simulink model "DOB_ros"  (R2017b)
settings: Solver=FixedStepAuto  StartTime=0.0  StopTime=inf  FixedStep=dt_ros  RelTol=1e-3
values from neighbouring files (symbols this model uses):
  a1 = @(vx, dphi) [0, 0, 0, 1]    [DOB_ros_adaptive_setup.m]    (also in DOB_ros_adaptive_w_kappa_setup.m = init)
  a2 = @(vx, dphi) [vx/cos(dphi)^2, 0, 1, ds]    [DOB_ros_adaptive_setup.m]    (also in DOB_ros_adaptive_w_kappa_setup.m = init)
  a3 = @(vx, dphi) [0, 0, -(Caf+Car)/(m*vx), -vx-(Caf*a-Car*b)/(m*vx)]    [DOB_ros_adaptive_setup.m]    (also in DOB_ros_adaptive_w_kappa_setup.m = init)
  b0 = init    [DOB_ros_adaptive_w_kappa_setup.m]
  b1 = init    [DOB_ros_adaptive_w_kappa_setup.m]    (also in DOB_ros_setup.m = 107.91)
  b2 = init    [DOB_ros_adaptive_w_kappa_setup.m]    (also in DOB_ros_setup.m = 71.28)
  b3 = Caf / m    (= 107.91)    [DOB_ros_adaptive_setup.m]    (also in DOB_ros_adaptive_w_kappa_setup.m = init)
  b4 = a * Caf / Iz    (= 71.28)    [DOB_ros_adaptive_setup.m]    (also in DOB_ros_adaptive_w_kappa_setup.m = init)
  b5 = init    [DOB_ros_adaptive_w_kappa_setup.m]
  Dd = single([Numc{1}(3:end) 0 0]/Numc{1}(3))    [DOB_ros_adaptive_setup.m]    (also in DOB_ros_adaptive_w_kappa_setup.m; DOB_ros_setup.m)
  Dn = single(Denc{1}/Numc{1}(3))    [DOB_ros_adaptive_setup.m]    (also in DOB_ros_adaptive_w_kappa_setup.m; DOB_ros_setup.m)
  dphi_list = -1:0.1:1    [DOB_ros_adaptive_w_kappa_setup.m]
  dt_ros = 0.02    [DOB_ros_adaptive_setup.m]    (also in DOB_ros_adaptive_w_kappa_setup.m; DOB_ros_setup.m)
  dt_ros_single = single(0.02)    [DOB_ros_adaptive_setup.m]    (also in DOB_ros_adaptive_w_kappa_setup.m; DOB_ros_setup.m)
  kappa_list = -0.02:0.005:0.02    [DOB_ros_adaptive_w_kappa_setup.m]
  kc11 = single(0.3)    [DOB_ros_adaptive_setup.m]    (also in DOB_ros_adaptive_w_kappa_setup.m = single(1); DOB_ros_setup.m = kc1)
  kc12 = single(1)    [DOB_ros_adaptive_setup.m]    (also in DOB_ros_adaptive_w_kappa_setup.m = single(0); DOB_ros_setup.m = 1)
  kc2 = single(0.25)    [DOB_ros_adaptive_setup.m]    (also in DOB_ros_adaptive_w_kappa_setup.m = single(0.5); DOB_ros_setup.m = single(0.1))
  steering_ratio = 14.8    [DOB_ros_adaptive_setup.m]    (also in DOB_ros_adaptive_w_kappa_setup.m; DOB_ros_setup.m)
  v_list = 1:0.2:20    [DOB_ros_adaptive_w_kappa_setup.m]
undefined symbols (not defined in the file or in its folder): DCancel, DEst, DQ, Enable, NQ, SteeringWheelAngleCmd, SteeringWheelAngleVelocity
libraries: robotlib x6, cstblocks x1
settings Model: Creator=chen_tang  LastModifiedBy=root
settings OptimizationCC: PassReuseOutputArgsThreshold=0  MaxStackSize=64
settings DebuggingCC: ParameterTunabilityLossMsg=error
settings HardwareCC: ProdBitPerPointer=32  ProdBitPerSizeT=32  ProdBitPerPtrDiffT=32  ProdLargestAtomicFloat=None  ProdIntDivRoundTo=Undefined  ProdEndianess=Unspecified  ProdWordSize=32  ProdHWDeviceType=Generic->Unspecified (assume 32-bit Generic)  UseEmbeddedCoderFeatures=off
settings SFSimCC: MATLABDynamicMemAlloc=off
settings RTWCC: SystemTargetFile=ert.tlc  HardwareBoard=Robot Operating System (ROS)  TemplateMakefile=ert_default_tmf  GenerateReport=on  Toolchain=Catkin  LaunchReport=on  TargetLang=C++
settings CodeAppCC: ForceParamTrailComments=on  OperatorAnnotations=on  StateflowObjectComments=on  MATLABSourceComments=on
settings ERTTargetCC: ERTCustomFileBanners=off  SupportContinuousTime=on  SupportNonInlinedSFcns=on  RemoveResetFunc=off  ModelStepFunctionPrototypeControlCompliant=off

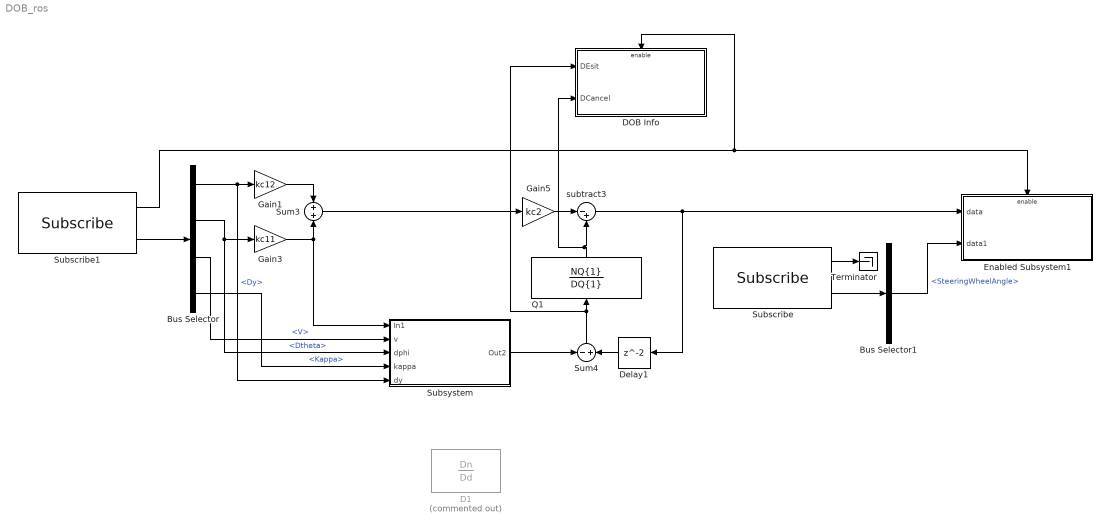
== system DOB_ros ==
  Bus Selector : BusSelector  OutputSignals=Dy,Dtheta,V,Kappa
  Bus Selector1 : BusSelector  OutputSignals=SteeringWheelAngle
  D1 : DiscreteTransferFcn  Commented=on  Numerator=Dn  Denominator=Dd  SampleTime=dt_ros
  DOB Info : Subsystem  TreatAsAtomicUnit=on
  Delay1 : Delay  InitialCondition=0  SampleTime=dt_ros
  Enabled Subsystem1 : Subsystem  TreatAsAtomicUnit=on
  Gain1 : Gain  Gain=kc12  OutDataTypeStr=single
  Gain3 : Gain  Gain=kc11  OutDataTypeStr=single
  Gain5 : Gain  Gain=kc2
  Q1 : DiscreteTransferFcn  Numerator=NQ{1}  Denominator=DQ{1}  SampleTime=dt_ros
  Subscribe : robotlib/Subscribe  SourceLibraryInfo=This block requires Robotics System Toolbox  topicSource=Specify your own  topic=/vehicle/steering_report  messageType=dbw_mkz_msgs/SteeringReport  sampleTime=-1  messageQueueLength=1
      settings: SourceProductBaseCode=RO
  Subscribe1 : robotlib/Subscribe  SourceLibraryInfo=This block requires Robotics System Toolbox  topicSource=Specify your own  topic=/tracking_info  messageType=controller/TrackingInfo  sampleTime=-1  messageQueueLength=1
      link override SourceBlock: ROSTopic=/tracking_info  ROSMessageType=controller/TrackingInfo  SLBusName=SL_Bus_DOB_ros_controller_TrackingInfo  ModelName=DOB_ros  BlockId=Sub_DOB_ros_174
      settings: SourceProductBaseCode=RO
  Subsystem : Subsystem
  Sum3 : Sum  Inputs=+|+  AccumDataTypeStr=single  OutDataTypeStr=single
  Sum4 : Sum  Inputs=-|+
  Terminator : Terminator
  subtract3 : Sum  Inputs=|-+  AccumDataTypeStr=single
  wires:
  Subscribe1/2 -> Bus Selector/1
  Gain3/1 -> Sum3/2, Subsystem/1(In1)
  Subscribe1/1 -> DOB Info/Enable, Enabled Subsystem1/Enable
  Bus Selector/2 -> Subsystem/3(dphi), Gain3/1  "<Dtheta>"
  Gain5/1 -> subtract3/1
  subtract3/1 -> Delay1/1, Enabled Subsystem1/1(data)
  Sum3/1 -> Gain5/1
  Subscribe/1 -> Terminator/1
  Subscribe/2 -> Bus Selector1/1
  Bus Selector1/1 -> Enabled Subsystem1/2(data1)  "<SteeringWheelAngle>"
  Delay1/1 -> Sum4/2
  Sum4/1 -> DOB Info/1(DEsit), Q1/1
  Subsystem/1(Out2) -> Sum4/1
  Q1/1 -> subtract3/2, DOB Info/2(DCancel)
  Bus Selector/1 -> Subsystem/5(dy), Gain1/1  "<Dy>"
  Gain1/1 -> Sum3/1
  Bus Selector/3 -> Subsystem/2(v)  "<V>"
  Bus Selector/4 -> Subsystem/4("kappa ")  "<Kappa>"

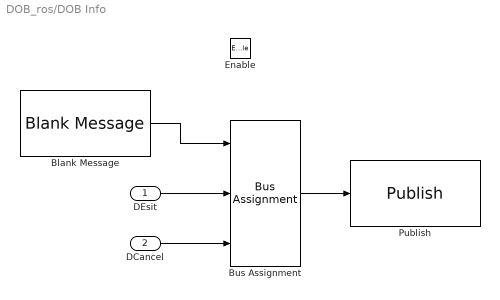
== system DOB_ros/DOB Info ==
  DEsit : Inport
  DCancel : Inport  Port=2
  Enable : EnablePort
  Blank Message : robotlib/Blank Message  SourceLibraryInfo=This block requires Robotics System Toolbox  messageType=controller/DobInfo  SampleTime=dt_ros
      settings: SourceProductBaseCode=RO
  Bus Assignment : BusAssignment  AssignedSignals=DEst,DCancel
  Publish : robotlib/Publish  SourceLibraryInfo=This block requires Robotics System Toolbox  topicSource=Specify your own  topic=/dob_info  messageType=controller/DobInfo  messageQueueLength=1
      settings: SourceProductBaseCode=RO
  wires:
  Bus Assignment/1 -> Publish/1
  Blank Message/1 -> Bus Assignment/1
  DEsit/1 -> Bus Assignment/2
  DCancel/1 -> Bus Assignment/3

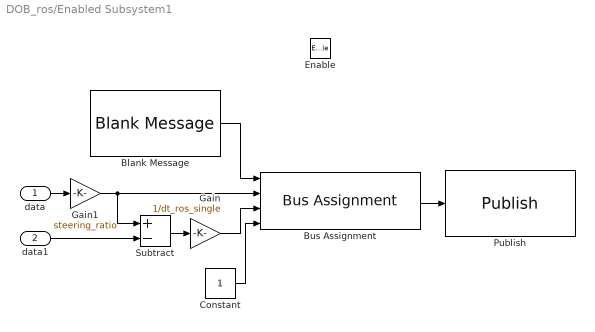
== system DOB_ros/Enabled Subsystem1 ==
  data : Inport  OutDataTypeStr=single
  data1 : Inport  Port=2  OutDataTypeStr=single
  Enable : EnablePort
  Blank Message : robotlib/Blank Message  SourceLibraryInfo=This block requires Robotics System Toolbox  messageType=dbw_mkz_msgs/SteeringCmd  SampleTime=dt_ros
      settings: SourceProductBaseCode=RO
  Bus Assignment : BusAssignment  AssignedSignals=SteeringWheelAngleCmd,SteeringWheelAngleVelocity,Enable
  Constant : Constant  OutDataTypeStr=boolean
  Gain : Gain  Gain=1/dt_ros_single  ParamDataTypeStr=single  OutDataTypeStr=single
  Gain1 : Gain  Gain=steering_ratio  ParamDataTypeStr=single  OutDataTypeStr=single
  Publish : robotlib/Publish  SourceLibraryInfo=This block requires Robotics System Toolbox  topicSource=Specify your own  topic=/vehicle/steering_cmd  messageType=dbw_mkz_msgs/SteeringCmd  messageQueueLength=1
      settings: SourceProductBaseCode=RO
  Subtract : Sum  Inputs=+-  AccumDataTypeStr=single  OutDataTypeStr=single
  wires:
  Bus Assignment/1 -> Publish/1
  data/1 -> Gain1/1
  Blank Message/1 -> Bus Assignment/1
  data1/1 -> Subtract/2
  Subtract/1 -> Gain/1
  Gain/1 -> Bus Assignment/3
  Gain1/1 -> Subtract/1, Bus Assignment/2
  Constant/1 -> Bus Assignment/4

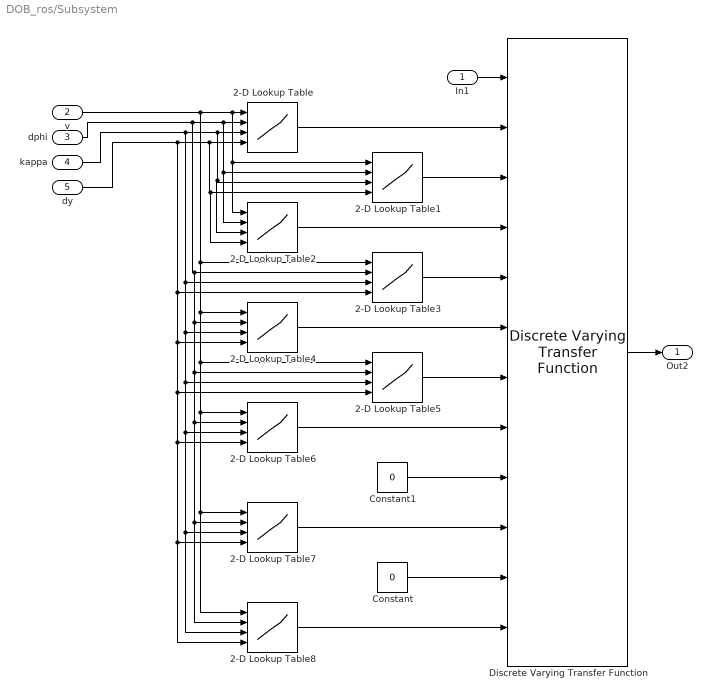
== system DOB_ros/Subsystem ==
  In1 : Inport
  v : Inport  Port=2
  dphi : Inport  Port=3
  "kappa " : Inport  Port=4
  dy : Inport  Port=5
  2-D Lookup Table : Lookup_n-D  NumberOfTableDimensions=4  BreakpointsForDimension1=v_list  BreakpointsForDimension2=dphi_list  BreakpointsForDimension3=kappa_list  BreakpointsForDimension4=dy_list  BeginIndexSearchUsingPreviousIndexResult=on  Table=b0  InternalRulePriority=Speed  OutDataTypeStr=single  RndMeth=Simplest  InputSameDT=on
  2-D Lookup Table1 : Lookup_n-D  NumberOfTableDimensions=4  BreakpointsForDimension1=v_list  BreakpointsForDimension2=dphi_list  BreakpointsForDimension3=kappa_list  BreakpointsForDimension4=dy_list  BeginIndexSearchUsingPreviousIndexResult=on  Table=a1  InternalRulePriority=Speed  OutDataTypeStr=single  RndMeth=Simplest  InputSameDT=on
  2-D Lookup Table2 : Lookup_n-D  NumberOfTableDimensions=4  BreakpointsForDimension1=v_list  BreakpointsForDimension2=dphi_list  BreakpointsForDimension3=kappa_list  BreakpointsForDimension4=dy_list  BeginIndexSearchUsingPreviousIndexResult=on  Table=b1  InternalRulePriority=Speed  OutDataTypeStr=single  RndMeth=Simplest  InputSameDT=on
  2-D Lookup Table3 : Lookup_n-D  NumberOfTableDimensions=4  BreakpointsForDimension1=v_list  BreakpointsForDimension2=dphi_list  BreakpointsForDimension3=kappa_list  BreakpointsForDimension4=dy_list  BeginIndexSearchUsingPreviousIndexResult=on  Table=a2  InternalRulePriority=Speed  OutDataTypeStr=single  RndMeth=Simplest  InputSameDT=on
  2-D Lookup Table4 : Lookup_n-D  NumberOfTableDimensions=4  BreakpointsForDimension1=v_list  BreakpointsForDimension2=dphi_list  BreakpointsForDimension3=kappa_list  BreakpointsForDimension4=dy_list  BeginIndexSearchUsingPreviousIndexResult=on  Table=b2  InternalRulePriority=Speed  OutDataTypeStr=single  RndMeth=Simplest  InputSameDT=on
  2-D Lookup Table5 : Lookup_n-D  NumberOfTableDimensions=4  BreakpointsForDimension1=v_list  BreakpointsForDimension2=dphi_list  BreakpointsForDimension3=kappa_list  BreakpointsForDimension4=dy_list  BeginIndexSearchUsingPreviousIndexResult=on  Table=a3  InternalRulePriority=Speed  OutDataTypeStr=single  RndMeth=Simplest  InputSameDT=on
  2-D Lookup Table6 : Lookup_n-D  NumberOfTableDimensions=4  BreakpointsForDimension1=v_list  BreakpointsForDimension2=dphi_list  BreakpointsForDimension3=kappa_list  BreakpointsForDimension4=dy_list  BeginIndexSearchUsingPreviousIndexResult=on  Table=b3  InternalRulePriority=Speed  OutDataTypeStr=single  RndMeth=Simplest  InputSameDT=on
  2-D Lookup Table7 : Lookup_n-D  NumberOfTableDimensions=4  BreakpointsForDimension1=v_list  BreakpointsForDimension2=dphi_list  BreakpointsForDimension3=kappa_list  BreakpointsForDimension4=dy_list  BeginIndexSearchUsingPreviousIndexResult=on  Table=b4  InternalRulePriority=Speed  OutDataTypeStr=single  RndMeth=Simplest  InputSameDT=on
  2-D Lookup Table8 : Lookup_n-D  NumberOfTableDimensions=4  BreakpointsForDimension1=v_list  BreakpointsForDimension2=dphi_list  BreakpointsForDimension3=kappa_list  BreakpointsForDimension4=dy_list  BeginIndexSearchUsingPreviousIndexResult=on  Table=b5  InternalRulePriority=Speed  OutDataTypeStr=single  RndMeth=Simplest  InputSameDT=on
  Constant : Constant  Value=0  OutDataTypeStr=single
  Constant1 : Constant  Value=0  OutDataTypeStr=single
  Discrete Varying Transfer Function : cstblocks/Linear Parameter Varying/Discrete Varying Transfer Function  N=5  Ts=dt_ros
      settings: SourceProductName=Control System Toolbox  SourceProductBaseCode=CT
  Out2 : Outport
  wires:
  Discrete Varying Transfer Function/1 -> Out2/1
  In1/1 -> Discrete Varying Transfer Function/1
  dphi/1 -> 2-D Lookup Table7/2, 2-D Lookup Table8/2, 2-D Lookup Table6/2, 2-D Lookup Table5/2, 2-D Lookup Table4/2, 2-D Lookup Table3/2, 2-D Lookup Table2/2, 2-D Lookup Table1/2, 2-D Lookup Table/2
  v/1 -> 2-D Lookup Table6/1, 2-D Lookup Table8/1, 2-D Lookup Table7/1, 2-D Lookup Table5/1, 2-D Lookup Table4/1, 2-D Lookup Table3/1, 2-D Lookup Table1/1, 2-D Lookup Table2/1, 2-D Lookup Table/1
  2-D Lookup Table/1 -> Discrete Varying Transfer Function/2
  2-D Lookup Table1/1 -> Discrete Varying Transfer Function/3
  2-D Lookup Table2/1 -> Discrete Varying Transfer Function/4
  2-D Lookup Table3/1 -> Discrete Varying Transfer Function/5
  Constant1/1 -> Discrete Varying Transfer Function/9
  Constant/1 -> Discrete Varying Transfer Function/11
  2-D Lookup Table7/1 -> Discrete Varying Transfer Function/10
  "kappa "/1 -> 2-D Lookup Table8/3, 2-D Lookup Table7/3, 2-D Lookup Table6/3, 2-D Lookup Table5/3, 2-D Lookup Table4/3, 2-D Lookup Table3/3, 2-D Lookup Table2/3, 2-D Lookup Table1/3, 2-D Lookup Table/3
  dy/1 -> 2-D Lookup Table8/4, 2-D Lookup Table7/4, 2-D Lookup Table6/4, 2-D Lookup Table5/4, 2-D Lookup Table4/4, 2-D Lookup Table3/4, 2-D Lookup Table2/4, 2-D Lookup Table1/4, 2-D Lookup Table/4
  2-D Lookup Table4/1 -> Discrete Varying Transfer Function/6
  2-D Lookup Table5/1 -> Discrete Varying Transfer Function/7
  2-D Lookup Table6/1 -> Discrete Varying Transfer Function/8
  2-D Lookup Table8/1 -> Discrete Varying Transfer Function/12
